simulink model "schwebekugel"  (R2015a)
settings: Solver=ode45  StartTime=0.0  StopTime=10.0  RelTol=1e-3
settings Model: Creator=leon  LastModifiedBy=leon

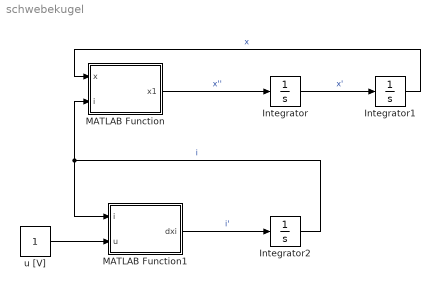
== system schwebekugel ==
  Integrator : Integrator
  Integrator1 : Integrator
  Integrator2 : Integrator
  MATLAB Function : MATLAB Function  TreatAsAtomicUnit=on
  MATLAB Function1 : MATLAB Function  TreatAsAtomicUnit=on
  u [V] : Constant
  wires:
  Integrator/1 -> Integrator1/1  "x'"
  MATLAB Function/1(x1) -> Integrator/1  "x''"
  Integrator1/1 -> MATLAB Function/1(x)  "x"
  MATLAB Function1/1(dxi) -> Integrator2/1  "i'"
  Integrator2/1 -> MATLAB Function/2(i), MATLAB Function1/1(i)  "i"
  u [V]/1 -> MATLAB Function1/2(u)

== matlab function schwebekugel/MATLAB Function1 ==
  data: i input; dxi output; u input
function dxi = fcn(i, u)
persistent R L;
R = 3;
L = 0.1;
dxi = (u - R * i)/L;

== matlab function schwebekugel/MATLAB Function ==
  data: x input; i input; x1 output
function x1 = fcn(x, i)
persistent m g C;
m = 0.025;
g = 9.81;
C = 5*10^-6;
mx = m * g - C * (i/x)^2;
x1 = mx/m;
